simulink model "PWM"  (R2020b)
settings: Solver=VariableStepAuto  StartTime=0.0  StopTime=10.0  RelTol=1e-3
model workspace (MAT data in the model file):
  Mf = 50
  mf = 1
  mf1 = 1
libraries: powerlib x14, powerlib_meascontrol x7, simulink x3
settings Model: ParameterArgumentNames=Mf  OrderedModelArguments=off  Creator=Yaipiti  LastModifiedBy=Yaipiti

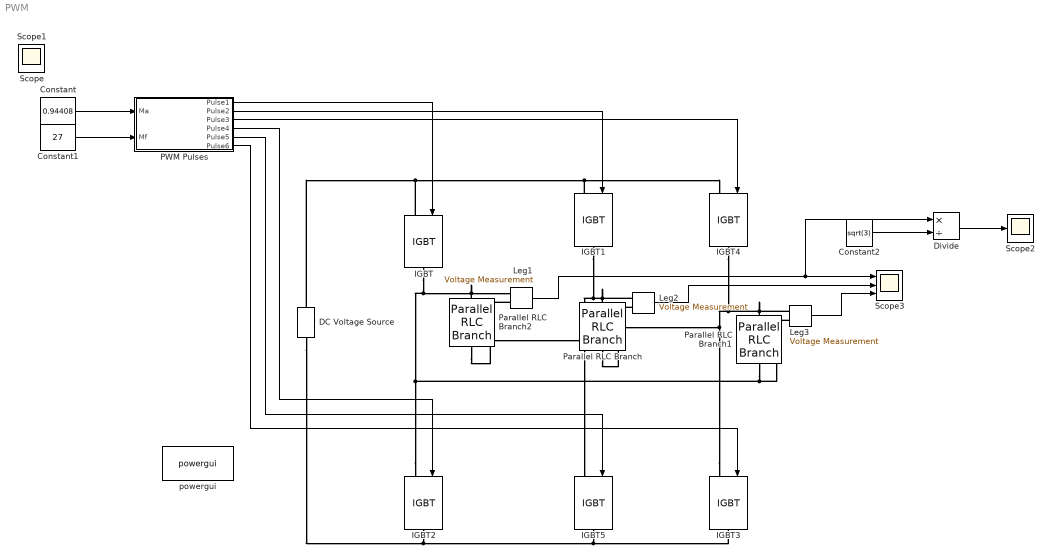
== system PWM ==
  Constant : Constant  Value=0.94408
  Constant1 : Constant  Value=27
  Constant2 : Constant  Value=sqrt(3)
  DC Voltage Source : powerlib/Electrical Sources/DC Voltage Source  Amplitude=360  Measurements=None
  Divide : Product  Inputs=*/
  IGBT{,1..5} (6 alike) : powerlib/Power Electronics/IGBT  Ron=0.001  Lon=0  Vf=1  Tf=1e-6  Tt=2e-6  IC=0  Rs=1e5  Cs=inf  Measurements=off
  Leg1 : powerlib/Measurements/Voltage Measurement  PhasorSimulation=off  OutputType=Complex  PSBequivalent=0
  Leg2 : powerlib/Measurements/Voltage Measurement  PhasorSimulation=off  OutputType=Complex  PSBequivalent=0
  Leg3 : powerlib/Measurements/Voltage Measurement  PhasorSimulation=off  OutputType=Complex  PSBequivalent=0
  PWM Pulses : Subsystem
  Parallel RLC Branch : powerlib/Elements/Parallel RLC Branch  LConnTagsString=a  RConnTagsString=__new0  BranchType=C  Resistance=1  Inductance=1e-3  SetiL0=off  InitialCurrent=0  Capacitance=0.002  Setx0=off  InitialVoltage=0  Measurements=None
  Parallel RLC Branch1 : powerlib/Elements/Parallel RLC Branch  LConnTagsString=a  RConnTagsString=__new0  BranchType=C  Resistance=1  Inductance=1e-3  SetiL0=off  InitialCurrent=0  Capacitance=0.002  Setx0=off  InitialVoltage=0  Measurements=None
  Parallel RLC Branch2 : powerlib/Elements/Parallel RLC Branch  LConnTagsString=a  RConnTagsString=__new0  BranchType=C  Resistance=1  Inductance=1e-3  SetiL0=off  InitialCurrent=0  Capacitance=0.002  Setx0=off  InitialVoltage=0  Measurements=None
  Scope2 : Scope
  Scope3 : Scope  NumInputPorts=3
  powergui : powerlib/powergui  Priority=1  SimulationMode=Continuous  SampleTime=50e-6  frequency=60  Iterations=50  frequencyindice=0  Pbase=100e6  ErrMax=1e-4  UnitsV=kV  UnitsW=MW  buscounter=0  FunctionMessages=off  echomessages=off  EnableUseOfTLC=off  CurrentSourceSwitches=off  DisableSnubberDevices=off  DisableRonSwitches=off  DisableVfSwitches=off  DisplayEquations=off  AutomaticDiscreteSolvers=off  SolverType=Tustin/Backward Euler (TBE)  Interpol=off  ExternalGateDelay=off  methode=off  Ts=100  x0status=blocks  SPID=on  SwTol=0  HookPort=off  NonlinearTolerance=1e-4  nMaxIteration=100  ContinueOnMaxIteration=off  RestoreLinks=warning  ResistiveCurrentMeasurement=off  Frange=[0:2:500]  Ylog=off  Xlog=on  ShowGrid=off  save=off  variable=ZData  structure=0  ZoomFFT=off  StartTime=0.0  cycles=1  DisplayStyle=1  fundamental=60  FreqAxis=off  MaxFrequency=1000  frequencyindicesteady=1  RmsSteady=1  display=off
  Scope : Scope
  Scope1 : Scope
  wires:
  Leg1/1 -> Divide/1, Scope3/1
  PWM Pulses/6(Pulse6) -> IGBT3/1
  PWM Pulses/5(Pulse5) -> IGBT5/1
  PWM Pulses/1(Pulse1) -> IGBT/1
  Leg2/1 -> Scope3/2
  PWM Pulses/2(Pulse2) -> IGBT1/1
  PWM Pulses/4(Pulse4) -> IGBT2/1
  PWM Pulses/3(Pulse3) -> IGBT4/1
  Leg3/1 -> Scope3/3
  Constant/1 -> PWM Pulses/1(Ma)
  Constant1/1 -> PWM Pulses/2(Mf)
  Constant2/1 -> Divide/2
  Divide/1 -> Scope2/1
  connections:
  IGBT4/LConn1 -- DC Voltage Source/RConn1 -- IGBT/LConn1 -- IGBT1/LConn1
  IGBT3/RConn1 -- DC Voltage Source/LConn1 -- IGBT2/RConn1 -- IGBT5/RConn1
  IGBT3/LConn1 -- Parallel RLC Branch/LConn1 -- Leg2/LConn2 -- Parallel RLC Branch1/RConn1 -- Leg3/LConn1 -- IGBT4/RConn1
  IGBT2/LConn1 -- Parallel RLC Branch1/LConn1 -- Leg3/LConn2 -- IGBT/RConn1 -- Parallel RLC Branch2/RConn1 -- Leg1/LConn1
  Leg1/LConn2 -- Parallel RLC Branch2/LConn1 -- Parallel RLC Branch/RConn1 -- Leg2/LConn1 -- IGBT1/RConn1 -- IGBT5/LConn1

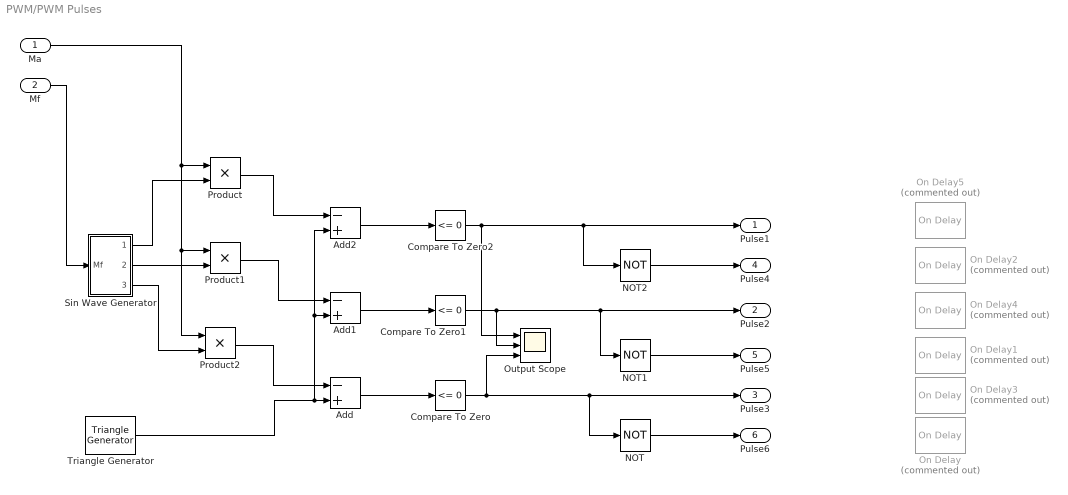
== system PWM/PWM Pulses ==
  Ma : Inport
  Mf : Inport  Port=2
  Add : Sum  Inputs=-+
  Add1 : Sum  Inputs=-+
  Add2 : Sum  Inputs=-+
  Compare To Zero : simulink/Logic and Bit Operations/Compare To Zero  relop=<=  OutDataTypeStr=uint8
  Compare To Zero1 : simulink/Logic and Bit Operations/Compare To Zero  relop=<=  OutDataTypeStr=uint8
  Compare To Zero2 : simulink/Logic and Bit Operations/Compare To Zero  relop=<=  OutDataTypeStr=uint8
  NOT : Logic  Operator=NOT  IconShape=distinctive  AllPortsSameDT=off  OutDataTypeStr=boolean
  NOT1 : Logic  Operator=NOT  IconShape=distinctive  AllPortsSameDT=off  OutDataTypeStr=boolean
  NOT2 : Logic  Operator=NOT  IconShape=distinctive  AllPortsSameDT=off  OutDataTypeStr=boolean
  On Delay{,1..5} (6 alike) : powerlib_meascontrol/Logic/On Delay  Commented=on  DelayType=On delay  delay=0.0007  ic=0  Ts=0
  Output Scope : Scope  NumInputPorts=3
  Product : Product
  Product1 : Product
  Product2 : Product
  Sin Wave Generator : Subsystem
  Triangle Generator : powerlib_meascontrol/Pulse & Signal Generators/Triangle Generator  Freq=60  Phase=90  Ts=0
  Pulse1 : Outport
  Pulse2 : Outport  Port=2
  Pulse3 : Outport  Port=3
  Pulse4 : Outport  Port=4
  Pulse5 : Outport  Port=5
  Pulse6 : Outport  Port=6
  wires:
  Compare To Zero1/1 -> Pulse2/1, NOT1/1, Output Scope/2
  Compare To Zero/1 -> Pulse3/1, NOT/1, Output Scope/3
  Add2/1 -> Compare To Zero2/1
  Triangle Generator/1 -> Add/2, Add2/2, Add1/2
  Add1/1 -> Compare To Zero1/1
  Product/1 -> Add2/1
  Product2/1 -> Add/1
  Add/1 -> Compare To Zero/1
  Compare To Zero2/1 -> Pulse1/1, NOT2/1, Output Scope/1
  NOT2/1 -> Pulse4/1
  NOT1/1 -> Pulse5/1
  NOT/1 -> Pulse6/1
  Product1/1 -> Add1/1
  Ma/1 -> Product2/1, Product1/1, Product/1
  Sin Wave Generator/1(Out1) -> Product/2
  Sin Wave Generator/2(Out2) -> Product1/2
  Sin Wave Generator/3(Out3) -> Product2/2
  Mf/1 -> Sin Wave Generator/1(Mf)

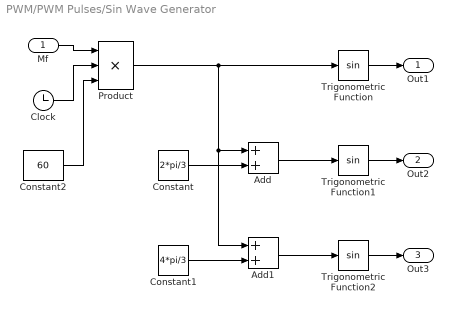
== system PWM/PWM Pulses/Sin Wave Generator ==
  Mf : Inport
  Add : Sum
  Add1 : Sum
  Clock : Clock
  Constant : Constant  Value=2*pi/3
  Constant1 : Constant  Value=4*pi/3
  Constant2 : Constant  Value=60
  Product : Product  Inputs=3
  Trigonometric Function : Trigonometry
  Trigonometric Function1 : Trigonometry
  Trigonometric Function2 : Trigonometry
  Out1 : Outport
  Out2 : Outport  Port=2
  Out3 : Outport  Port=3
  wires:
  Clock/1 -> Product/2
  Mf/1 -> Product/1
  Trigonometric Function/1 -> Out1/1
  Product/1 -> Add/1, Add1/1, Trigonometric Function/1
  Trigonometric Function2/1 -> Out3/1
  Trigonometric Function1/1 -> Out2/1
  Constant2/1 -> Product/3
  Add1/1 -> Trigonometric Function2/1
  Add/1 -> Trigonometric Function1/1
  Constant/1 -> Add/2
  Constant1/1 -> Add1/2
